simulink subsystem "PowerSystemRef"  (R2024b)
settings: Solver=VariableStepAuto  StartTime=0.0  StopTime=10.0  RelTol=1e-3
undefined symbols (not defined in the file): ess, geom, mot, mot2, mot3, mot4, propel, propel2, propel3, propel4, pxf_diagram_options, SimIn, tc, tc2, tc3, tc4
libraries: simulink x10, slpidlib x5
(part 10 of 10)

== system PowerSystemRef/powerplant/mot4/ctrl/cmd/mot4_ctrl_cmd_map_Pelec_funTW_volt_in/avoid zero output ==
  In1 : Inport
  Constant : Constant  Value=eps
  Switch1 : Switch  Criteria=u2 ~= 0  SaturateOnIntegerOverflow=off  InputSameDT=off
  Out1 : Outport
  wires:
  In1/1 -> Switch1/2, Switch1/1
  Constant/1 -> Switch1/3
  Switch1/1 -> Out1/1

== system PowerSystemRef/powerplant/mot4/ctrl/cstr/mot4_ctrl_cstr_map_Pelec_funTW_volt_in/Continuous torque - Prop ==
  input x : Inport
  map : Lookup  InputValues=x  Table=map
  map limits on x : Saturate  UpperLimit=max(x)  LowerLimit=min(x)
  output : Outport
  wires:
  map limits on x/1 -> map/1
  map/1 -> output/1
  input x/1 -> map limits on x/1

== system PowerSystemRef/powerplant/mot4/ctrl/cstr/mot4_ctrl_cstr_map_Pelec_funTW_volt_in/Continuous torque _regen ==
  input x : Inport
  map : Lookup  InputValues=x  Table=map
  map limits on x : Saturate  UpperLimit=max(x)  LowerLimit=min(x)
  output : Outport
  wires:
  map limits on x/1 -> map/1
  map/1 -> output/1
  input x/1 -> map limits on x/1

== system PowerSystemRef/powerplant/mot4/ctrl/cstr/mot4_ctrl_cstr_map_Pelec_funTW_volt_in/Peak torque - Prop ==
  input x : Inport
  map : Lookup  InputValues=x  Table=map
  map limits on x : Saturate  UpperLimit=max(x)  LowerLimit=min(x)
  output : Outport
  wires:
  map limits on x/1 -> map/1
  map/1 -> output/1
  input x/1 -> map limits on x/1

== system PowerSystemRef/powerplant/mot4/ctrl/cstr/mot4_ctrl_cstr_map_Pelec_funTW_volt_in/Peak torque _regen ==
  input x : Inport
  map : Lookup  InputValues=x  Table=map
  map limits on x : Saturate  UpperLimit=max(x)  LowerLimit=min(x)
  output : Outport
  wires:
  map limits on x/1 -> map/1
  map/1 -> output/1
  input x/1 -> map limits on x/1

== system PowerSystemRef/powerplant/mot4/ctrl/dmd/mot4_ctrl_dmd_uas/Determine_Required_Motor_RPS ==
  Prop_D : Inport
  rho : Inport  Port=2
  P : Inport  Port=3
  CPpoly : Inport  Port=4
  Algebraic Constraint : AlgebraicConstraint  InitialGuess=100
  Demux : Demux  Outputs=2
  Fcn : Fcn  Expr=u(4)*u(6)^4 + u(5)*u(6)^3 - u(3)/u(2)/u(1)^5
  MATLAB Function : MATLAB Function  Commented=on  TreatAsAtomicUnit=on
  Mux : Mux  Inputs=6
  RPS_req : Outport  VectorParamsAs1DForOutWhenUnconnected=off
  wires:
  Fcn/1 -> Algebraic Constraint/1
  Algebraic Constraint/1 -> Mux/6, RPS_req/1  "RPS_req"
  Mux/1 -> Fcn/1
  CPpoly/1 -> Demux/1
  Demux/2 -> Mux/5
  Demux/1 -> Mux/4
  Prop_D/1 -> Mux/1
  P/1 -> Mux/3
  rho/1 -> Mux/2

== system PowerSystemRef/powerplant/mot4/ctrl/dmd/mot4_ctrl_dmd_uas/mot_propel_plant_init_eff_map ==
  input x : Inport
  map : Lookup  InputValues=x  Table=map
  map limits on x : Saturate  UpperLimit=max(x)  LowerLimit=min(x)
  output : Outport  VectorParamsAs1DForOutWhenUnconnected=off
  wires:
  input x/1 -> map limits on x/1
  map/1 -> output/1
  map limits on x/1 -> map/1

== system PowerSystemRef/powerplant/mot4/plant/mot4_plant_map_Pelec_funTW_volt_in/max torque /Cont trq max - Prop ==
  input x : Inport
  map : Lookup  InputValues=x  Table=map
  map limits on x : Saturate  UpperLimit=max(x)  LowerLimit=min(x)
  output : Outport
  wires:
  input x/1 -> map limits on x/1
  map/1 -> output/1
  map limits on x/1 -> map/1

== system PowerSystemRef/powerplant/mot4/plant/mot4_plant_map_Pelec_funTW_volt_in/max torque /Cont trq max - Regen ==
  input x : Inport
  map : Lookup  InputValues=x  Table=map
  map limits on x : Saturate  UpperLimit=max(x)  LowerLimit=min(x)
  output : Outport
  wires:
  map limits on x/1 -> map/1
  map/1 -> output/1
  input x/1 -> map limits on x/1

== system PowerSystemRef/powerplant/mot4/plant/mot4_plant_map_Pelec_funTW_volt_in/max torque /Heat index ==
  note: Heat index calculation
  note: to avoid spikes
      |  due to
      | div by zero
  cont torque : Inport
  torque : Inport  Port=2
  Abs : Abs
  Divide : Subsystem  mask(Divide){}
      mask Display: disp('Divide')
  Heat Energy Factor : Integrator  InitialCondition=-0.3  LimitOutput=on  UpperSaturationLimit=1  LowerSaturationLimit=-0.3
  Heating Constant : Gain  Gain=0.3/mot4.plant.init.t_max_trq  SaturateOnIntegerOverflow=on  OutDataTypeStr=Inherit: Same as input  ParamDataTypeStr=Inherit: Same as input
  Saturation : Saturate  UpperLimit=1  LowerLimit=0
  Saturation1 : Saturate  UpperLimit=10  LowerLimit=0
  Sum : Sum  Inputs=+-  InputSameDT=on  SaturateOnIntegerOverflow=on  OutDataTypeStr=Inherit: Same as first input
  motor inertia (Nms^2\rad)5 : Constant
  Heat index : Outport
  wires:
  Saturation1/1 -> Sum/1
  torque/1 -> Divide/1(numerator)
  Heat Energy Factor/1 -> Saturation/1
  Heating Constant/1 -> Heat Energy Factor/1
  Sum/1 -> Heating Constant/1
  Divide/1(quotient) -> Abs/1
  motor inertia (Nms^2\rad)5/1 -> Sum/2
  Saturation/1 -> Heat index/1
  Abs/1 -> Saturation1/1
  cont torque/1 -> Divide/2(denominator)

== system PowerSystemRef/powerplant/mot4/plant/mot4_plant_map_Pelec_funTW_volt_in/max torque /Peak trq max - Prop ==
  input x : Inport
  map : Lookup  InputValues=x  Table=map
  map limits on x : Saturate  UpperLimit=max(x)  LowerLimit=min(x)
  output : Outport
  wires:
  map limits on x/1 -> map/1
  map/1 -> output/1
  input x/1 -> map limits on x/1

== system PowerSystemRef/powerplant/mot4/plant/mot4_plant_map_Pelec_funTW_volt_in/max torque /Peak trq max - Regen ==
  input x : Inport
  map : Lookup  InputValues=x  Table=map
  map limits on x : Saturate  UpperLimit=max(x)  LowerLimit=min(x)
  output : Outport
  wires:
  input x/1 -> map limits on x/1
  map/1 -> output/1
  map limits on x/1 -> map/1

== system PowerSystemRef/powerplant/propel/plant/propel_plant_uas/Propeller_CP/propel_plant_init_CP_CT_map ==
  input x : Inport
  map : Lookup  InputValues=x  Table=map
  map limits on x : Saturate  UpperLimit=max(x)  LowerLimit=min(x)
  output : Outport  VectorParamsAs1DForOutWhenUnconnected=off
  wires:
  map limits on x/1 -> map/1
  map/1 -> output/1
  input x/1 -> map limits on x/1

== system PowerSystemRef/powerplant/propel/plant/propel_plant_uas/Thrust_Generated/propel_plant_init_CP_CT_map ==
  input x : Inport
  map : Lookup  InputValues=x  Table=map
  map limits on x : Saturate  UpperLimit=max(x)  LowerLimit=min(x)
  output : Outport  VectorParamsAs1DForOutWhenUnconnected=off
  wires:
  input x/1 -> map limits on x/1
  map/1 -> output/1
  map limits on x/1 -> map/1

== system PowerSystemRef/powerplant/propel/plant/propel_plant_uas/Total_Moment/Moment_due_to_eng_position ==
  Vec 1 : Inport
  Vec 2 : Inport  Port=2
  Mux : Mux  Inputs=2
  Mux1 : Mux  Inputs=3
  i axis : Fcn  Expr=u[6]*u[2] - u[5]*u[3]
  j axis : Fcn  Expr=u[4]*u[3] - u[6]*u[1]
  k axis : Fcn  Expr=u[5]*u[1] - u[4]*u[2]
  X Prod : Outport  VectorParamsAs1DForOutWhenUnconnected=off
  wires:
  Mux1/1 -> X Prod/1
  k axis/1 -> Mux1/3
  i axis/1 -> Mux1/1
  j axis/1 -> Mux1/2
  Mux/1 -> i axis/1, k axis/1, j axis/1
  Vec 1/1 -> Mux/1
  Vec 2/1 -> Mux/2

== system PowerSystemRef/powerplant/propel2/plant/propel2_plant_uas/Propeller_CP/propel_plant_init_CP_CT_map ==
  input x : Inport
  map : Lookup  InputValues=x  Table=map
  map limits on x : Saturate  UpperLimit=max(x)  LowerLimit=min(x)
  output : Outport  VectorParamsAs1DForOutWhenUnconnected=off
  wires:
  map limits on x/1 -> map/1
  map/1 -> output/1
  input x/1 -> map limits on x/1

== system PowerSystemRef/powerplant/propel2/plant/propel2_plant_uas/Thrust_Generated/propel_plant_init_CP_CT_map ==
  input x : Inport
  map : Lookup  InputValues=x  Table=map
  map limits on x : Saturate  UpperLimit=max(x)  LowerLimit=min(x)
  output : Outport  VectorParamsAs1DForOutWhenUnconnected=off
  wires:
  input x/1 -> map limits on x/1
  map/1 -> output/1
  map limits on x/1 -> map/1

== system PowerSystemRef/powerplant/propel2/plant/propel2_plant_uas/Total_Moment/Moment_due_to_eng_position ==
  Vec 1 : Inport
  Vec 2 : Inport  Port=2
  Mux : Mux  Inputs=2
  Mux1 : Mux  Inputs=3
  i axis : Fcn  Expr=u[6]*u[2] - u[5]*u[3]
  j axis : Fcn  Expr=u[4]*u[3] - u[6]*u[1]
  k axis : Fcn  Expr=u[5]*u[1] - u[4]*u[2]
  X Prod : Outport  VectorParamsAs1DForOutWhenUnconnected=off
  wires:
  Mux1/1 -> X Prod/1
  k axis/1 -> Mux1/3
  i axis/1 -> Mux1/1
  j axis/1 -> Mux1/2
  Mux/1 -> i axis/1, k axis/1, j axis/1
  Vec 1/1 -> Mux/1
  Vec 2/1 -> Mux/2

== system PowerSystemRef/powerplant/propel3/plant/propel3_plant_uas/Propeller_CP/propel_plant_init_CP_CT_map ==
  input x : Inport
  map : Lookup  InputValues=x  Table=map
  map limits on x : Saturate  UpperLimit=max(x)  LowerLimit=min(x)
  output : Outport  VectorParamsAs1DForOutWhenUnconnected=off
  wires:
  map limits on x/1 -> map/1
  map/1 -> output/1
  input x/1 -> map limits on x/1

== system PowerSystemRef/powerplant/propel3/plant/propel3_plant_uas/Thrust_Generated/propel_plant_init_CP_CT_map ==
  input x : Inport
  map : Lookup  InputValues=x  Table=map
  map limits on x : Saturate  UpperLimit=max(x)  LowerLimit=min(x)
  output : Outport  VectorParamsAs1DForOutWhenUnconnected=off
  wires:
  input x/1 -> map limits on x/1
  map/1 -> output/1
  map limits on x/1 -> map/1

== system PowerSystemRef/powerplant/propel3/plant/propel3_plant_uas/Total_Moment/Moment_due_to_eng_position ==
  Vec 1 : Inport
  Vec 2 : Inport  Port=2
  Mux : Mux  Inputs=2
  Mux1 : Mux  Inputs=3
  i axis : Fcn  Expr=u[6]*u[2] - u[5]*u[3]
  j axis : Fcn  Expr=u[4]*u[3] - u[6]*u[1]
  k axis : Fcn  Expr=u[5]*u[1] - u[4]*u[2]
  X Prod : Outport  VectorParamsAs1DForOutWhenUnconnected=off
  wires:
  Mux1/1 -> X Prod/1
  k axis/1 -> Mux1/3
  i axis/1 -> Mux1/1
  j axis/1 -> Mux1/2
  Mux/1 -> i axis/1, k axis/1, j axis/1
  Vec 1/1 -> Mux/1
  Vec 2/1 -> Mux/2

== system PowerSystemRef/powerplant/propel4/plant/propel4_plant_uas/Propeller_CP/propel_plant_init_CP_CT_map ==
  input x : Inport
  map : Lookup  InputValues=x  Table=map
  map limits on x : Saturate  UpperLimit=max(x)  LowerLimit=min(x)
  output : Outport  VectorParamsAs1DForOutWhenUnconnected=off
  wires:
  map limits on x/1 -> map/1
  map/1 -> output/1
  input x/1 -> map limits on x/1

== system PowerSystemRef/powerplant/propel4/plant/propel4_plant_uas/Thrust_Generated/propel_plant_init_CP_CT_map ==
  input x : Inport
  map : Lookup  InputValues=x  Table=map
  map limits on x : Saturate  UpperLimit=max(x)  LowerLimit=min(x)
  output : Outport  VectorParamsAs1DForOutWhenUnconnected=off
  wires:
  input x/1 -> map limits on x/1
  map/1 -> output/1
  map limits on x/1 -> map/1

== system PowerSystemRef/powerplant/propel4/plant/propel4_plant_uas/Total_Moment/Moment_due_to_eng_position ==
  Vec 1 : Inport
  Vec 2 : Inport  Port=2
  Mux : Mux  Inputs=2
  Mux1 : Mux  Inputs=3
  i axis : Fcn  Expr=u[6]*u[2] - u[5]*u[3]
  j axis : Fcn  Expr=u[4]*u[3] - u[6]*u[1]
  k axis : Fcn  Expr=u[5]*u[1] - u[4]*u[2]
  X Prod : Outport  VectorParamsAs1DForOutWhenUnconnected=off
  wires:
  Mux1/1 -> X Prod/1
  k axis/1 -> Mux1/3
  i axis/1 -> Mux1/1
  j axis/1 -> Mux1/2
  Mux/1 -> i axis/1, k axis/1, j axis/1
  Vec 1/1 -> Mux/1
  Vec 2/1 -> Mux/2

== system PowerSystemRef/powerplant/tc/plant/tc_plant_map_trqloss_funTW/Torque calculation/Blending (state dependent) ==
  Input : Inport
  Control (state) : Inport  Port=2
  Linear spline : Fcn  Expr=(u<xl)*yl + (xl<=u)*(u<xc)*((yc-yl)*(u-xl)/(xc-xl)+yl) + (xc<=u)*(u<xr)*((yc-yr)*(u-xr)/(xc-xr)+yr) + (xr<=u)*yr
  Product2 : Product  InputSameDT=on  SaturateOnIntegerOverflow=on  OutDataTypeStr=Inherit: Same as first input
  Output : Outport
  wires:
  Input/1 -> Product2/1
  Linear spline/1 -> Product2/2
  Product2/1 -> Output/1
  Control (state)/1 -> Linear spline/1

== system PowerSystemRef/powerplant/tc/plant/tc_plant_map_trqloss_funTW/Torque calculation/trq losses ==
  Rows : Inport
  Cols : Inport  Port=2
  Look-Up Table (2-D) : Lookup2D  RowIndex=x  ColumnIndex=y  Table=t
  Out1 : Outport
  wires:
  Look-Up Table (2-D)/1 -> Out1/1
  Cols/1 -> Look-Up Table (2-D)/2
  Rows/1 -> Look-Up Table (2-D)/1

== system PowerSystemRef/powerplant/tc2/plant/tc2_plant_map_trqloss_funTW/Torque calculation/Blending (state dependent) ==
  Input : Inport
  Control (state) : Inport  Port=2
  Linear spline : Fcn  Expr=(u<xl)*yl + (xl<=u)*(u<xc)*((yc-yl)*(u-xl)/(xc-xl)+yl) + (xc<=u)*(u<xr)*((yc-yr)*(u-xr)/(xc-xr)+yr) + (xr<=u)*yr
  Product2 : Product  InputSameDT=on  SaturateOnIntegerOverflow=on  OutDataTypeStr=Inherit: Same as first input
  Output : Outport
  wires:
  Input/1 -> Product2/1
  Linear spline/1 -> Product2/2
  Product2/1 -> Output/1
  Control (state)/1 -> Linear spline/1

== system PowerSystemRef/powerplant/tc2/plant/tc2_plant_map_trqloss_funTW/Torque calculation/trq losses ==
  Rows : Inport
  Cols : Inport  Port=2
  Look-Up Table (2-D) : Lookup2D  RowIndex=x  ColumnIndex=y  Table=t
  Out1 : Outport
  wires:
  Look-Up Table (2-D)/1 -> Out1/1
  Cols/1 -> Look-Up Table (2-D)/2
  Rows/1 -> Look-Up Table (2-D)/1

== system PowerSystemRef/powerplant/tc3/plant/tc3_plant_map_trqloss_funTW/Torque calculation/Blending (state dependent) ==
  Input : Inport
  Control (state) : Inport  Port=2
  Linear spline : Fcn  Expr=(u<xl)*yl + (xl<=u)*(u<xc)*((yc-yl)*(u-xl)/(xc-xl)+yl) + (xc<=u)*(u<xr)*((yc-yr)*(u-xr)/(xc-xr)+yr) + (xr<=u)*yr
  Product2 : Product  InputSameDT=on  SaturateOnIntegerOverflow=on  OutDataTypeStr=Inherit: Same as first input
  Output : Outport
  wires:
  Input/1 -> Product2/1
  Linear spline/1 -> Product2/2
  Product2/1 -> Output/1
  Control (state)/1 -> Linear spline/1

== system PowerSystemRef/powerplant/tc3/plant/tc3_plant_map_trqloss_funTW/Torque calculation/trq losses ==
  Rows : Inport
  Cols : Inport  Port=2
  Look-Up Table (2-D) : Lookup2D  RowIndex=x  ColumnIndex=y  Table=t
  Out1 : Outport
  wires:
  Look-Up Table (2-D)/1 -> Out1/1
  Cols/1 -> Look-Up Table (2-D)/2
  Rows/1 -> Look-Up Table (2-D)/1

== system PowerSystemRef/powerplant/tc4/plant/tc4_plant_map_trqloss_funTW/Torque calculation/Blending (state dependent) ==
  Input : Inport
  Control (state) : Inport  Port=2
  Linear spline : Fcn  Expr=(u<xl)*yl + (xl<=u)*(u<xc)*((yc-yl)*(u-xl)/(xc-xl)+yl) + (xc<=u)*(u<xr)*((yc-yr)*(u-xr)/(xc-xr)+yr) + (xr<=u)*yr
  Product2 : Product  InputSameDT=on  SaturateOnIntegerOverflow=on  OutDataTypeStr=Inherit: Same as first input
  Output : Outport
  wires:
  Input/1 -> Product2/1
  Linear spline/1 -> Product2/2
  Product2/1 -> Output/1
  Control (state)/1 -> Linear spline/1

== system PowerSystemRef/powerplant/tc4/plant/tc4_plant_map_trqloss_funTW/Torque calculation/trq losses ==
  Rows : Inport
  Cols : Inport  Port=2
  Look-Up Table (2-D) : Lookup2D  RowIndex=x  ColumnIndex=y  Table=t
  Out1 : Outport
  wires:
  Look-Up Table (2-D)/1 -> Out1/1
  Cols/1 -> Look-Up Table (2-D)/2
  Rows/1 -> Look-Up Table (2-D)/1

== system PowerSystemRef/powerplant/ess (battery)/ctrl/ess_ctrl_pngv_map_anl_PI_cstr/PI controller for maximal charge power and current1/PI Ratio Calculator (curr) /non-zero division1 ==
  note: original idea from Phil Sharer - ANL
      | original formula: u[1]\(u[2]+eps)*(u[2]!=0)
      | changes done by Gerald ZINI (dgey) - ANL (05\02\2001)
  note: (u[2]==0) is true then returns 1, thus (u[2]+(u[2]==0)) is equal to 0+1=1
  note: if u[2] == 0, then output == 0:
  note: (u[2]!=0) is false then returns 0
  note: and finally, the expression is: (u[1] \ 1) * 0 = 0
  note: (u[2]==0) is false then returns 0, thus (u[2]+(u[2]==0)) is equal to u[2]+0=u[2]
  note: if u[2] != 0, then output == u[1]\u[2]:
  note: (u[2]!=0) is true then returns 1
  note: and finally, the expression is: (u[1] \ u[2]) * 1 = u[1] \ u[2]
  In1 : Inport
  In2 : Inport  Port=2
  Fcn : Fcn  Expr=u[1]/(u[2]+(u[2]==0))*(u[2]!=0)
  Mux : Mux  Inputs=2
  Out1 : Outport
  wires:
  Mux/1 -> Fcn/1
  In1/1 -> Mux/1
  Fcn/1 -> Out1/1
  In2/1 -> Mux/2

== system PowerSystemRef/powerplant/ess (battery)/ctrl/ess_ctrl_pngv_map_anl_PI_cstr/PI controller for maximal charge power and current1/PI Ratio Calculator (curr) 1/non-zero division1 ==
  note: original idea from Phil Sharer - ANL
      | original formula: u[1]\(u[2]+eps)*(u[2]!=0)
      | changes done by Gerald ZINI (dgey) - ANL (05\02\2001)
  note: (u[2]==0) is true then returns 1, thus (u[2]+(u[2]==0)) is equal to 0+1=1
  note: if u[2] == 0, then output == 0:
  note: (u[2]!=0) is false then returns 0
  note: and finally, the expression is: (u[1] \ 1) * 0 = 0
  note: (u[2]==0) is false then returns 0, thus (u[2]+(u[2]==0)) is equal to u[2]+0=u[2]
  note: if u[2] != 0, then output == u[1]\u[2]:
  note: (u[2]!=0) is true then returns 1
  note: and finally, the expression is: (u[1] \ u[2]) * 1 = u[1] \ u[2]
  In1 : Inport
  In2 : Inport  Port=2
  Fcn : Fcn  Expr=u[1]/(u[2]+(u[2]==0))*(u[2]!=0)
  Mux : Mux  Inputs=2
  Out1 : Outport
  wires:
  Mux/1 -> Fcn/1
  In1/1 -> Mux/1
  Fcn/1 -> Out1/1
  In2/1 -> Mux/2

== system PowerSystemRef/powerplant/ess (battery)/ctrl/ess_ctrl_pngv_map_anl_PI_cstr/PI controller for maximal discharge power and current1/PI Ratio Calculator (curr) /non-zero division1 ==
  note: and finally, the expression is: (u[1] \ u[2]) * 1 = u[1] \ u[2]
  note: (u[2]!=0) is true then returns 1
  note: if u[2] != 0, then output == u[1]\u[2]:
  note: (u[2]==0) is false then returns 0, thus (u[2]+(u[2]==0)) is equal to u[2]+0=u[2]
  note: and finally, the expression is: (u[1] \ 1) * 0 = 0
  note: (u[2]!=0) is false then returns 0
  note: if u[2] == 0, then output == 0:
  note: (u[2]==0) is true then returns 1, thus (u[2]+(u[2]==0)) is equal to 0+1=1
  note: original idea from Phil Sharer - ANL
      | original formula: u[1]\(u[2]+eps)*(u[2]!=0)
      | changes done by Gerald ZINI (dgey) - ANL (05\02\2001)
  In1 : Inport
  In2 : Inport  Port=2
  Fcn : Fcn  Expr=u[1]/(u[2]+(u[2]==0))*(u[2]!=0)
  Mux : Mux  Inputs=2
  Out1 : Outport
  wires:
  In2/1 -> Mux/2
  Fcn/1 -> Out1/1
  In1/1 -> Mux/1
  Mux/1 -> Fcn/1

== system PowerSystemRef/powerplant/ess (battery)/ctrl/ess_ctrl_pngv_map_anl_PI_cstr/PI controller for maximal discharge power and current1/PI Ratio Calculator (curr) 1/non-zero division1 ==
  note: original idea from Phil Sharer - ANL
      | original formula: u[1]\(u[2]+eps)*(u[2]!=0)
      | changes done by Gerald ZINI (dgey) - ANL (05\02\2001)
  note: (u[2]==0) is true then returns 1, thus (u[2]+(u[2]==0)) is equal to 0+1=1
  note: if u[2] == 0, then output == 0:
  note: (u[2]!=0) is false then returns 0
  note: and finally, the expression is: (u[1] \ 1) * 0 = 0
  note: (u[2]==0) is false then returns 0, thus (u[2]+(u[2]==0)) is equal to u[2]+0=u[2]
  note: if u[2] != 0, then output == u[1]\u[2]:
  note: (u[2]!=0) is true then returns 1
  note: and finally, the expression is: (u[1] \ u[2]) * 1 = u[1] \ u[2]
  In1 : Inport
  In2 : Inport  Port=2
  Fcn : Fcn  Expr=u[1]/(u[2]+(u[2]==0))*(u[2]!=0)
  Mux : Mux  Inputs=2
  Out1 : Outport
  wires:
  Mux/1 -> Fcn/1
  In1/1 -> Mux/1
  Fcn/1 -> Out1/1
  In2/1 -> Mux/2

== system PowerSystemRef/powerplant/ess (battery)1/ctrl/ess_ctrl_pngv_map_anl_PI_cstr/PI controller for maximal charge power and current1/PI Ratio Calculator (curr) /non-zero division1 ==
  note: and finally, the expression is: (u[1] \ u[2]) * 1 = u[1] \ u[2]
  note: (u[2]!=0) is true then returns 1
  note: if u[2] != 0, then output == u[1]\u[2]:
  note: (u[2]==0) is false then returns 0, thus (u[2]+(u[2]==0)) is equal to u[2]+0=u[2]
  note: and finally, the expression is: (u[1] \ 1) * 0 = 0
  note: (u[2]!=0) is false then returns 0
  note: if u[2] == 0, then output == 0:
  note: (u[2]==0) is true then returns 1, thus (u[2]+(u[2]==0)) is equal to 0+1=1
  note: original idea from Phil Sharer - ANL
      | original formula: u[1]\(u[2]+eps)*(u[2]!=0)
      | changes done by Gerald ZINI (dgey) - ANL (05\02\2001)
  In1 : Inport
  In2 : Inport  Port=2
  Fcn : Fcn  Expr=u[1]/(u[2]+(u[2]==0))*(u[2]!=0)
  Mux : Mux  Inputs=2
  Out1 : Outport
  wires:
  In2/1 -> Mux/2
  Fcn/1 -> Out1/1
  In1/1 -> Mux/1
  Mux/1 -> Fcn/1

== system PowerSystemRef/powerplant/ess (battery)1/ctrl/ess_ctrl_pngv_map_anl_PI_cstr/PI controller for maximal charge power and current1/PI Ratio Calculator (curr) 1/non-zero division1 ==
  note: and finally, the expression is: (u[1] \ u[2]) * 1 = u[1] \ u[2]
  note: (u[2]!=0) is true then returns 1
  note: if u[2] != 0, then output == u[1]\u[2]:
  note: (u[2]==0) is false then returns 0, thus (u[2]+(u[2]==0)) is equal to u[2]+0=u[2]
  note: and finally, the expression is: (u[1] \ 1) * 0 = 0
  note: (u[2]!=0) is false then returns 0
  note: if u[2] == 0, then output == 0:
  note: (u[2]==0) is true then returns 1, thus (u[2]+(u[2]==0)) is equal to 0+1=1
  note: original idea from Phil Sharer - ANL
      | original formula: u[1]\(u[2]+eps)*(u[2]!=0)
      | changes done by Gerald ZINI (dgey) - ANL (05\02\2001)
  In1 : Inport
  In2 : Inport  Port=2
  Fcn : Fcn  Expr=u[1]/(u[2]+(u[2]==0))*(u[2]!=0)
  Mux : Mux  Inputs=2
  Out1 : Outport
  wires:
  In2/1 -> Mux/2
  Fcn/1 -> Out1/1
  In1/1 -> Mux/1
  Mux/1 -> Fcn/1

== system PowerSystemRef/powerplant/ess (battery)1/ctrl/ess_ctrl_pngv_map_anl_PI_cstr/PI controller for maximal discharge power and current1/PI Ratio Calculator (curr) /non-zero division1 ==
  note: original idea from Phil Sharer - ANL
      | original formula: u[1]\(u[2]+eps)*(u[2]!=0)
      | changes done by Gerald ZINI (dgey) - ANL (05\02\2001)
  note: (u[2]==0) is true then returns 1, thus (u[2]+(u[2]==0)) is equal to 0+1=1
  note: if u[2] == 0, then output == 0:
  note: (u[2]!=0) is false then returns 0
  note: and finally, the expression is: (u[1] \ 1) * 0 = 0
  note: (u[2]==0) is false then returns 0, thus (u[2]+(u[2]==0)) is equal to u[2]+0=u[2]
  note: if u[2] != 0, then output == u[1]\u[2]:
  note: (u[2]!=0) is true then returns 1
  note: and finally, the expression is: (u[1] \ u[2]) * 1 = u[1] \ u[2]
  In1 : Inport
  In2 : Inport  Port=2
  Fcn : Fcn  Expr=u[1]/(u[2]+(u[2]==0))*(u[2]!=0)
  Mux : Mux  Inputs=2
  Out1 : Outport
  wires:
  Mux/1 -> Fcn/1
  In1/1 -> Mux/1
  Fcn/1 -> Out1/1
  In2/1 -> Mux/2

== system PowerSystemRef/powerplant/ess (battery)1/ctrl/ess_ctrl_pngv_map_anl_PI_cstr/PI controller for maximal discharge power and current1/PI Ratio Calculator (curr) 1/non-zero division1 ==
  note: and finally, the expression is: (u[1] \ u[2]) * 1 = u[1] \ u[2]
  note: (u[2]!=0) is true then returns 1
  note: if u[2] != 0, then output == u[1]\u[2]:
  note: (u[2]==0) is false then returns 0, thus (u[2]+(u[2]==0)) is equal to u[2]+0=u[2]
  note: and finally, the expression is: (u[1] \ 1) * 0 = 0
  note: (u[2]!=0) is false then returns 0
  note: if u[2] == 0, then output == 0:
  note: (u[2]==0) is true then returns 1, thus (u[2]+(u[2]==0)) is equal to 0+1=1
  note: original idea from Phil Sharer - ANL
      | original formula: u[1]\(u[2]+eps)*(u[2]!=0)
      | changes done by Gerald ZINI (dgey) - ANL (05\02\2001)
  In1 : Inport
  In2 : Inport  Port=2
  Fcn : Fcn  Expr=u[1]/(u[2]+(u[2]==0))*(u[2]!=0)
  Mux : Mux  Inputs=2
  Out1 : Outport
  wires:
  In2/1 -> Mux/2
  Fcn/1 -> Out1/1
  In1/1 -> Mux/1
  Mux/1 -> Fcn/1

== system PowerSystemRef/powerplant/mot/plant/mot_plant_map_Pelec_funTW_volt_in/max torque /Heat index/Divide ==
  note: Take care of
      | division by 0
  numerator : Inport
  denominator : Inport  Port=2
  Fcn : Fcn  Expr=u[1] / ( u[2] + eps*(u[2]==0) )
  Mux : Mux  Inputs=2
  quotient : Outport
  wires:
  Mux/1 -> Fcn/1
  numerator/1 -> Mux/1
  Fcn/1 -> quotient/1
  denominator/1 -> Mux/2

== system PowerSystemRef/powerplant/mot2/plant/mot2_plant_map_Pelec_funTW_volt_in/max torque /Heat index/Divide ==
  note: Take care of
      | division by 0
  numerator : Inport
  denominator : Inport  Port=2
  Fcn : Fcn  Expr=u[1] / ( u[2] + eps*(u[2]==0) )
  Mux : Mux  Inputs=2
  quotient : Outport
  wires:
  Mux/1 -> Fcn/1
  numerator/1 -> Mux/1
  Fcn/1 -> quotient/1
  denominator/1 -> Mux/2

== system PowerSystemRef/powerplant/mot3/plant/mot3_plant_map_Pelec_funTW_volt_in/max torque /Heat index/Divide ==
  note: Take care of
      | division by 0
  numerator : Inport
  denominator : Inport  Port=2
  Fcn : Fcn  Expr=u[1] / ( u[2] + eps*(u[2]==0) )
  Mux : Mux  Inputs=2
  quotient : Outport
  wires:
  Mux/1 -> Fcn/1
  numerator/1 -> Mux/1
  Fcn/1 -> quotient/1
  denominator/1 -> Mux/2

== system PowerSystemRef/powerplant/mot4/plant/mot4_plant_map_Pelec_funTW_volt_in/max torque /Heat index/Divide ==
  note: Take care of
      | division by 0
  numerator : Inport
  denominator : Inport  Port=2
  Fcn : Fcn  Expr=u[1] / ( u[2] + eps*(u[2]==0) )
  Mux : Mux  Inputs=2
  quotient : Outport
  wires:
  Mux/1 -> Fcn/1
  numerator/1 -> Mux/1
  Fcn/1 -> quotient/1
  denominator/1 -> Mux/2

== matlab function PowerSystemRef/mot/ctrl/dmd/mot_ctrl_dmd_uas/Determine_Required_Motor_RPS/MATLAB Function ==
  data: Prop_D input; RPS_req output; rho input; P input; CPpoly input
function RPS_req = fcn(Prop_D, rho, P, CPpoly)

n = roots([CPpoly(1), CPpoly(2), 0, 0, -P/rho/Prop_D^5]);
% Roots returns complex numbers by default, also Simulink doesn't like when
% the output is variable size, so have to make these contraptions to exctact
% the right root, usually between 0 and 300 rps.
n = real(n) + imag(n);
rp = n(0<n & n<300);
if isempty(rp)
    RPS_req = 0;
else
    RPS_req = rp(1);
end

== matlab function PowerSystemRef/powerplant/mot/ctrl/dmd/mot_ctrl_dmd_uas/Determine_Required_Motor_RPS/MATLAB Function ==
  data: Prop_D input; RPS_req output; rho input; P input; CPpoly input
function RPS_req = fcn(Prop_D, rho, P, CPpoly)

n = roots([CPpoly(1), CPpoly(2), 0, 0, -P/rho/Prop_D^5]);
% Roots returns complex numbers by default, also Simulink doesn't like when
% the output is variable size, so have to make these contraptions to exctact
% the right root, usually between 0 and 300 rps.
n = real(n) + imag(n);
rp = n(0<n & n<300);
if isempty(rp)
    RPS_req = 0;
else
    RPS_req = rp(1);
end

== matlab function PowerSystemRef/powerplant/mot3/ctrl/dmd/mot3_ctrl_dmd_uas/Determine_Required_Motor_RPS/MATLAB Function ==
  data: Prop_D input; RPS_req output; rho input; P input; CPpoly input
function RPS_req = fcn(Prop_D, rho, P, CPpoly)

n = roots([CPpoly(1), CPpoly(2), 0, 0, -P/rho/Prop_D^5]);
% Roots returns complex numbers by default, also Simulink doesn't like when
% the output is variable size, so have to make these contraptions to exctact
% the right root, usually between 0 and 300 rps.
n = real(n) + imag(n);
rp = n(0<n & n<300);
if isempty(rp)
    RPS_req = 0;
else
    RPS_req = rp(1);
end

== matlab function PowerSystemRef/powerplant/mot4/ctrl/dmd/mot4_ctrl_dmd_uas/Determine_Required_Motor_RPS/MATLAB Function ==
  data: Prop_D input; RPS_req output; rho input; P input; CPpoly input
function RPS_req = fcn(Prop_D, rho, P, CPpoly)

n = roots([CPpoly(1), CPpoly(2), 0, 0, -P/rho/Prop_D^5]);
% Roots returns complex numbers by default, also Simulink doesn't like when
% the output is variable size, so have to make these contraptions to exctact
% the right root, usually between 0 and 300 rps.
n = real(n) + imag(n);
rp = n(0<n & n<300);
if isempty(rp)
    RPS_req = 0;
else
    RPS_req = rp(1);
end

== matlab function PowerSystemRef/powerplant/mot2/ctrl/dmd/mot2_ctrl_dmd_uas/Determine_Required_Motor_RPS/MATLAB Function ==
  data: Prop_D input; RPS_req output; rho input; P input; CPpoly input
function RPS_req = fcn(Prop_D, rho, P, CPpoly)

n = roots([CPpoly(1), CPpoly(2), 0, 0, -P/rho/Prop_D^5]);
% Roots returns complex numbers by default, also Simulink doesn't like when
% the output is variable size, so have to make these contraptions to exctact
% the right root, usually between 0 and 300 rps.
n = real(n) + imag(n);
rp = n(0<n & n<300);
if isempty(rp)
    RPS_req = 0;
else
    RPS_req = rp(1);
end
